simulink model "modello_dinamico"  (R2022b)
settings: Solver=VariableStepAuto  StartTime=0.0  StopTime=40  RelTol=1e-3
model workspace (MAT data in the model file):
  a = 1
values from neighbouring files (symbols this model uses):
  dt = log_vars.dt    [EKF.m]    (also in EKF_for_smoother.m; UKF.m; getJacobian.m; plot_filters.m)
  L = P*H'*inv(S)    [EKF.m]    (also in EKF_for_smoother.m; UKF.m = Pxy*(S)^(-1))
undefined symbols (not defined in the file or in its folder): b, IPy, IPz, rp, sigbuilder_block, std_dev_db, std_dev_dx, std_dev_phi_dot, std_dev_psi, std_dev_tau_phi, std_dev_tau_psi, X_start
settings Model: Creator=alexi  LastModifiedBy=franc

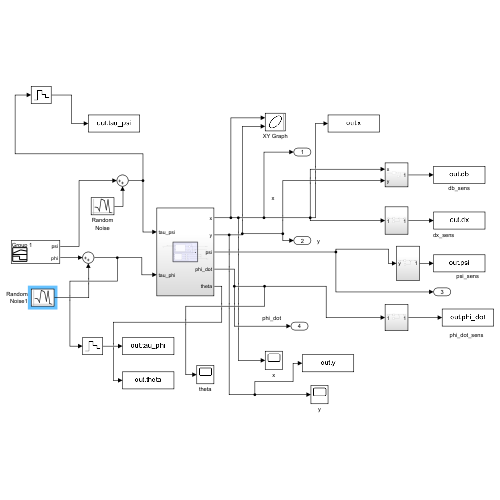
[thumbnail: Simulink's stored preview of the top-level diagram]
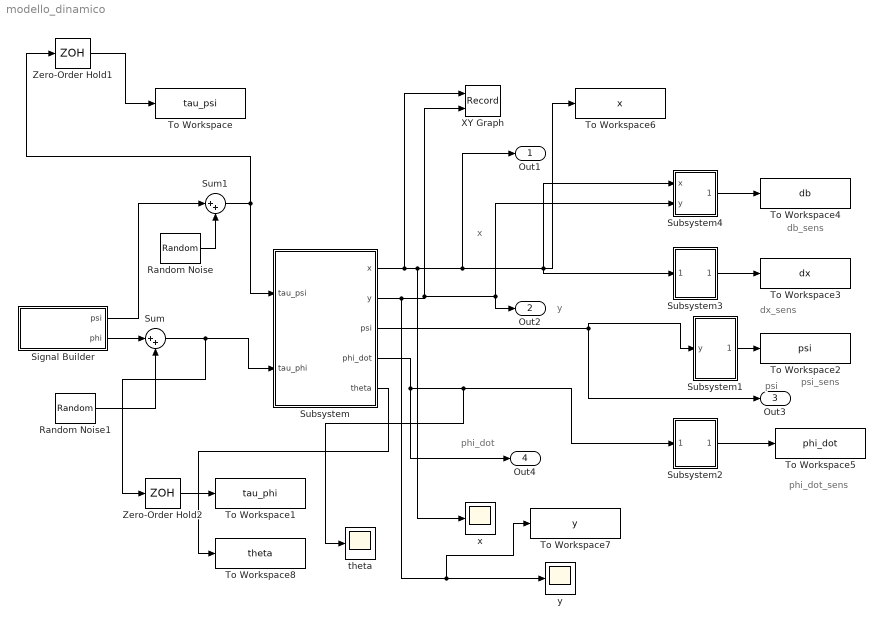
== system modello_dinamico ==
  note: db_sens
  note: dx_sens
  note: phi_dot
  note: phi_dot_sens
  note: psi_sens
  note: x
  note: y
  note: psi
  Random Noise : RandomNumber  Variance=(std_dev_tau_psi)^2  SampleTime=dt
  Random Noise1 : RandomNumber  Variance=(std_dev_tau_phi)^2  SampleTime=dt
  Signal Builder : Subsystem  Tag=STV Subsys  LoadFcn=sigbuilder_block('load');  StartFcn=sigbuilder_block('start');  StopFcn=sigbuilder_block('stop');  ClipboardFcn=sigbuilder_block('clipboard');  mask(Sigbuilder block){tuvar=[0:10]}
      mask help: Simulink:masks:SigbuilderBlock_MD
      mask init:
      | if ~strcmp(get_param(bdroot(gcbh),'SimulationStatus'),'stopped') tuvar = sigbuilder_block('maskInit'); end
      settings: CopyFcn=sigbuilder_block('copy');  DeleteFcn=sigbuilder_block('delete');  ModelCloseFcn=sigbuilder_block('modelClose');  PreSaveFcn=sigbuilder_block('preSave');  PauseFcn=sigbuilder_block('pause');  ContinueFcn=sigbuilder_block('continue');  NameChangeFcn=sigbuilder_block('namechange');  OpenFcn=sigbuilder_block('open',[5.4 30 1141.2 522.6 ]);  CloseFcn=sigbuilder_block('close');
      mask Display: plot(0, 0, 100, 100,[2, 2, 32, 32, 2], [68, 8, 8, 68, 68],[32, 2], [38, 38], [32, 19, 2],[53, 60, 44], [32, 17, 17, 2],[16, 16, 31, 31]);txt = getActiveGroup(gcbh);text(2, 100, txt,'verticalAlignment', 'top');
  Subsystem : Subsystem
  Subsystem1 : Subsystem
  Subsystem2 : Subsystem
  Subsystem3 : Subsystem
  Subsystem4 : Subsystem
  Sum : Sum  Inputs=|++
  Sum1 : Sum  Inputs=|++
  To Workspace : ToWorkspace  VariableName=tau_psi  SampleTime=-1
  To Workspace1 : ToWorkspace  VariableName=tau_phi  SampleTime=-1
  To Workspace2 : ToWorkspace  VariableName=psi  SampleTime=dt
  To Workspace3 : ToWorkspace  VariableName=dx  SampleTime=dt
  To Workspace4 : ToWorkspace  VariableName=db  SampleTime=dt
  To Workspace5 : ToWorkspace  VariableName=phi_dot  SampleTime=dt
  To Workspace6 : ToWorkspace  VariableName=x  SampleTime=-1
  To Workspace7 : ToWorkspace  VariableName=y  SampleTime=-1
  To Workspace8 : ToWorkspace  VariableName=theta  SampleTime=dt
  XY Graph : Record  FileSettingsInternal="{\"entries\":[{\"content\":{\"excelSettings\":{\"content\":{},\"type\":\"Streamout.ExcelSettings\"}},\"type\":\"Streamout.FileSettingStorage\",\"uuid\":\"96c72458-5053-4086-97b9-ba21e0ac0ac8\"}],\"packageUris\":[\"http://schema.mathworks.com/mf0/streamout_blocks/R2020a\"],\"version\":\"1.0\"}"  Layout=[1 1]  SignalsInternal="{\"entries\":[{\"content\":{\"signals\":[{\"content\":{\"blockPath\":[\"modello_dinamico/XY Graph\"],\"channel\":[],\"dimensions\":[1],\"domain\":\"modello_dinamico/XY Graph\",\"lineColor\":\"#a2142f\",\"plots\":[1],\"port\":1,\"sid\":[\"\"],\"signalID\":3214,\"signalName\":\"Subsystem:1\"},\"type\":\"RecordBlkView.Signal\",\"uuid\":\"133771aa-af28-4f69-9bdc-0cc03fee71db\"},{\"content\":{\"blockPath\":[\"modello_dinamico/XY Graph\"],\"channel\":[],\"dimensions\":[1],\"domain\":\"modello_dinamico/XY Graph\",\"lineColor\":\"#139fff\",\"plots\":[1],\"port\":2,\"sid\":[\"\"],\"signalID\":3218,\"signalName\":\"Subsystem:2\"},\"type\":\"RecordBlkView.Signal\",\"uuid\":\"00cd0381-8dc5-4a36-8ceb-bd6dd47d7666\"}]},\"type\":\"RecordBlkView.InputSignals\",\"uuid\":\"b5728904-0e35-463e-9761-cc6a3a068bd3\"}],\"packageUris\":[\"http://schema.mathworks.com/mf0/streamout_blocks/R2020a\"],\"version\":\"1.0\"}"  VisualizationBindings="{\"xyplotplugin\":{\"info\":[{\"series\":[{\"bindingParametersList\":[{\"parameter\":\"X-Axis\",\"signalID\":3214,\"signalName\":\"Subsystem:1\"},{\"parameter\":\"Y-Axis\",\"signalID\":3218,\"signalName\":\"Subsystem:2\"}],\"seriesID\":61188}],\"subplotID\":1}]}}"  CompatibilityTag=XY
  Zero-Order Hold1 : ZeroOrderHold  SampleTime=dt
  Zero-Order Hold2 : ZeroOrderHold  SampleTime=dt
  theta : Scope
  x : Scope
  y : Scope
  Out1 : Outport
  Out2 : Outport  Port=2
  Out3 : Outport  Port=3
  Out4 : Outport  Port=4
  wires:
  Subsystem/2(y) -> y/1, To Workspace7/1, Out2/1, Subsystem4/2(y), XY Graph/2
  Subsystem1/1(Output) -> To Workspace2/1
  Subsystem/4(phi_dot) -> Out4/1, theta/1, Subsystem2/1(In1)
  Subsystem4/1(Out1) -> To Workspace4/1
  Signal Builder/2(phi) -> Sum/1
  Sum/1 -> Zero-Order Hold2/1, Subsystem/2(tau_phi)
  Signal Builder/1(psi) -> Sum1/1
  Sum1/1 -> Zero-Order Hold1/1, Subsystem/1(tau_psi)
  Zero-Order Hold2/1 -> To Workspace1/1
  Zero-Order Hold1/1 -> To Workspace/1
  Subsystem3/1(Output) -> To Workspace3/1
  Subsystem2/1(Output) -> To Workspace5/1
  Subsystem/1(x) -> To Workspace6/1, Subsystem4/1(x), Subsystem3/1(In1), Out1/1, x/1, XY Graph/1
  Subsystem/3(psi) -> Subsystem1/1(y), Out3/1
  Subsystem/5(theta) -> To Workspace8/1
  Random Noise/1 -> Sum1/2
  Random Noise1/1 -> Sum/2

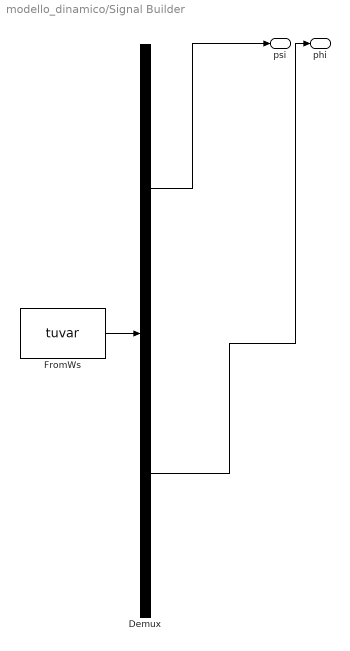
== system modello_dinamico/Signal Builder ==
  Demux : Demux  Tag=STV Demux  Outputs=2
      settings: DisplayOption=none
  FromWs : FromWorkspace  Tag=STV FromWs  VariableName=tuvar
      SigBuilderData=|
      | common.afterFinalStr = 'Extrapolate'
      | common.sampleTime = 0
      | dataSet.timeRange = [0 40]
      | dataSet.name = 'Group 1'
      | sbobj.Groups.Name = 'Group 1'
      | sbobj.Groups.Signals(1).Name = 'psi'
      | sbobj.Groups.Signals(1).XData = [0 5 5 5.5 5.5 40]
      | sbobj.Groups.Signals(1).YData = [0 0 0.005 0.005 0 0]
      | sbobj.Groups.Signals(2).Name = 'phi'
      | sbobj.Groups.Signals(2).XData = [0 7.83 40]
      | sbobj.Groups.Signals(2).YData = [0 0.05 0.05]
      | sbobj.Groups.TimeRange = [0 40]
  psi : Outport  Tag=STV Outport
  phi : Outport  Tag=STV Outport  Port=2
  wires:
  Demux/1 -> psi/1
  FromWs/1 -> Demux/1
  Demux/2 -> phi/1

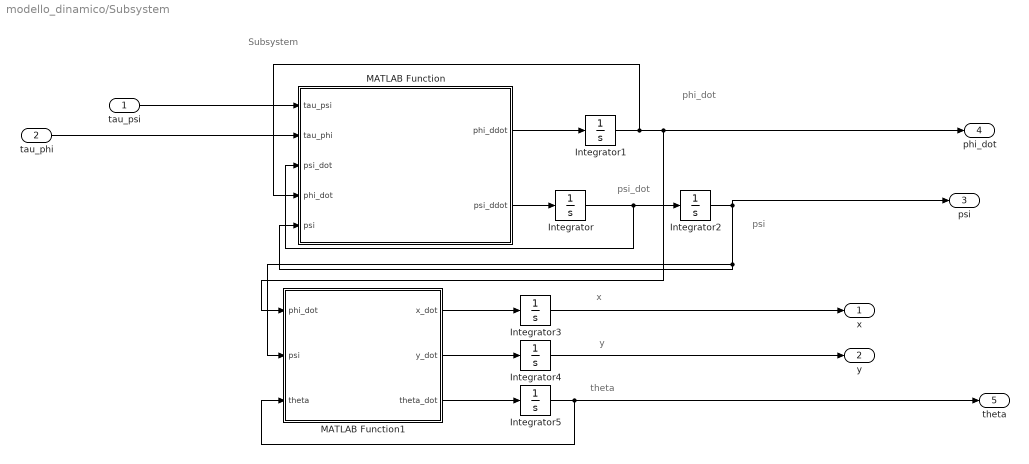
== system modello_dinamico/Subsystem ==
  note: Subsystem
  note: phi_dot
  note: psi_dot
  note: psi
  note: theta
  note: y
  note: x
  tau_psi : Inport
  tau_phi : Inport  Port=2
  Integrator : Integrator  InitialCondition=X_start(6)
  Integrator1 : Integrator  InitialCondition=X_start(4)
  Integrator2 : Integrator  InitialCondition=X_start(5)
  Integrator3 : Integrator  InitialCondition=X_start(1)
  Integrator4 : Integrator  InitialCondition=X_start(2)
  Integrator5 : Integrator  InitialCondition=X_start(3)
  MATLAB Function : MATLAB Function  TreatAsAtomicUnit=on
  MATLAB Function1 : MATLAB Function  TreatAsAtomicUnit=on
  x : Outport
  y : Outport  Port=2
  psi : Outport  Port=3
  phi_dot : Outport  Port=4
  theta : Outport  Port=5
  wires:
  Integrator3/1 -> x/1
  Integrator4/1 -> y/1
  Integrator2/1 -> MATLAB Function1/2(psi), MATLAB Function/5(psi), psi/1
  Integrator1/1 -> MATLAB Function1/1(phi_dot), phi_dot/1, MATLAB Function/4(phi_dot)
  MATLAB Function/1(phi_ddot) -> Integrator1/1
  MATLAB Function1/1(x_dot) -> Integrator3/1
  tau_psi/1 -> MATLAB Function/1(tau_psi)
  Integrator/1 -> Integrator2/1, MATLAB Function/3(psi_dot)
  MATLAB Function/2(psi_ddot) -> Integrator/1
  MATLAB Function1/2(y_dot) -> Integrator4/1
  tau_phi/1 -> MATLAB Function/2(tau_phi)
  MATLAB Function1/3(theta_dot) -> Integrator5/1
  Integrator5/1 -> theta/1, MATLAB Function1/3(theta)

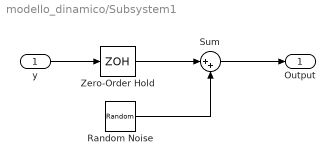
== system modello_dinamico/Subsystem1 ==
  y : Inport
  Random Noise : RandomNumber  Variance=(std_dev_psi)^2  SampleTime=dt
  Sum : Sum  Inputs=|++
  Zero-Order Hold : ZeroOrderHold  SampleTime=dt
  Output : Outport
  wires:
  Random Noise/1 -> Sum/2
  y/1 -> Zero-Order Hold/1
  Zero-Order Hold/1 -> Sum/1
  Sum/1 -> Output/1

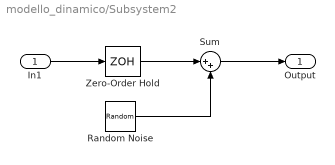
== system modello_dinamico/Subsystem2 ==
  In1 : Inport
  Random Noise : RandomNumber  Variance=(std_dev_phi_dot)^2  SampleTime=dt
  Sum : Sum  Inputs=|++
  Zero-Order Hold : ZeroOrderHold  SampleTime=dt
  Output : Outport
  wires:
  Random Noise/1 -> Sum/2
  In1/1 -> Zero-Order Hold/1
  Zero-Order Hold/1 -> Sum/1
  Sum/1 -> Output/1

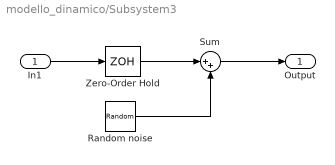
== system modello_dinamico/Subsystem3 ==
  In1 : Inport
  Random noise : RandomNumber  Variance=(std_dev_dx)^2  SampleTime=dt
  Sum : Sum  Inputs=|++
  Zero-Order Hold : ZeroOrderHold  SampleTime=dt
  Output : Outport
  wires:
  Random noise/1 -> Sum/2
  In1/1 -> Zero-Order Hold/1
  Zero-Order Hold/1 -> Sum/1
  Sum/1 -> Output/1

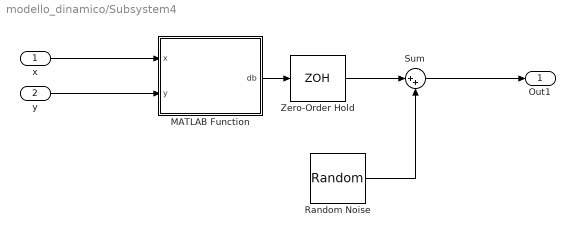
== system modello_dinamico/Subsystem4 ==
  x : Inport
  y : Inport  Port=2
  MATLAB Function : MATLAB Function  TreatAsAtomicUnit=on
  Random Noise : RandomNumber  Variance=(std_dev_db)^2  SampleTime=dt
  Sum : Sum  Inputs=|++
  Zero-Order Hold : ZeroOrderHold  SampleTime=dt
  Out1 : Outport
  wires:
  MATLAB Function/1(db) -> Zero-Order Hold/1
  y/1 -> MATLAB Function/2(y)
  Zero-Order Hold/1 -> Sum/1
  x/1 -> MATLAB Function/1(x)
  Random Noise/1 -> Sum/2
  Sum/1 -> Out1/1

== matlab function modello_dinamico/Subsystem/MATLAB Function1 ==
  data: phi_dot input; psi input; theta input; x_dot output; y_dot output; theta_dot output; rp parameter; L parameter
function [x_dot,y_dot,theta_dot] = KinematicModel(phi_dot,psi,theta,rp,L)
%impostare a,b,c come parametri da prendere dal workspace
x_dot = rp*phi_dot*cos(theta)*cos(psi);
y_dot = rp*phi_dot*sin(theta)*cos(psi);
theta_dot= -rp*phi_dot*sin(psi)/L;

== matlab function modello_dinamico/Subsystem/MATLAB Function ==
  data: tau_psi input; phi_ddot output; tau_phi input; psi_dot input; phi_dot input; psi input; psi_ddot output; a parameter; b parameter; rp parameter; L parameter; IPy parameter size=1; IPz parameter
function [phi_ddot,psi_ddot] = DynamicModel(tau_psi,tau_phi,psi_dot,phi_dot,psi,a, b,rp, L, IPy, IPz)
B=[a*rp^2*cos(psi)^2+b*(rp/L)^2*sin(psi)^2+IPy -IPz*(rp/L)*sin(psi);-IPz*(rp/L)*sin(psi) IPz];
C=[(rp^2*b/L^2-a*rp^2)*cos(psi)*sin(psi)*psi_dot*phi_dot;-IPz*rp/L*cos(psi)*psi_dot*phi_dot];
tau = [tau_phi;tau_psi];
M = inv(B)*(tau-C);
phi_ddot=M(1);
psi_ddot=M(2);

== matlab function modello_dinamico/Subsystem4/MATLAB Function ==
  data: x input; db output; y input; D parameter
function db = calculate_db(x,y,D)
db = sqrt(y^2+(D-x)^2);
